simulink library "csc_cnt_attitude_control_lib_diag"  (R2015b)
settings: Solver=ode45  StartTime=0.0  StopTime=10.0  RelTol=1e-3
undefined symbols (not defined in the file or in its folder): csc_cnt_dt, gdn_altitude_transition_free_drift_landing, gdn_altitude_transition_free_drift_takeoff
libraries: util_quat_lib x3, util_common_lib x2, util_info_lib x1, util_extra_lib x1, csc_ppc_phase_plane_ctrl_lib_diag x1, csu_iqf_inertial_quat_feedback_lib x1
settings Model: Creator=ianmga  LastModifiedBy=jimkaidy
settings DataIOCC: SaveFormat=Array  SignalLoggingSaveFormat=ModelDataLogs
settings OptimizationCC: ExpressionDepthLimit=2147483647
settings DebuggingCC: UnderspecifiedInitializationDetection=Classic  MergeDetectMultiDrivingBlocksExec=none  SolverPrmCheckMsg=warning  FcnCallInpInsideContextMsg=UseLocalSettings  StateNameClashWarn=warning
settings HardwareCC: ProdBitPerPointer=32  ProdLargestAtomicFloat=None  ProdIntDivRoundTo=Undefined  ProdEndianess=Unspecified  ProdWordSize=32  ProdHWDeviceType=32-bit Generic
settings GRTTargetCC: GeneratePreprocessorConditionals=Disable all  CombineOutputUpdateFcns=off  GRTInterface=on
settings ConfigComp: CovModelRefEnable=Off  CovSFcnEnable=off

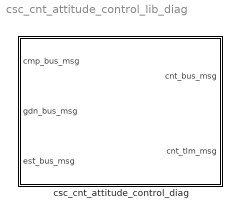
== system csc_cnt_attitude_control_lib_diag ==
  csc_cnt_attitude_control_diag : Subsystem  Tag=OFSW; MDL_TICK=GDN_BUS_MSG  TreatAsAtomicUnit=on  SystemSampleTime=csc_cnt_dt

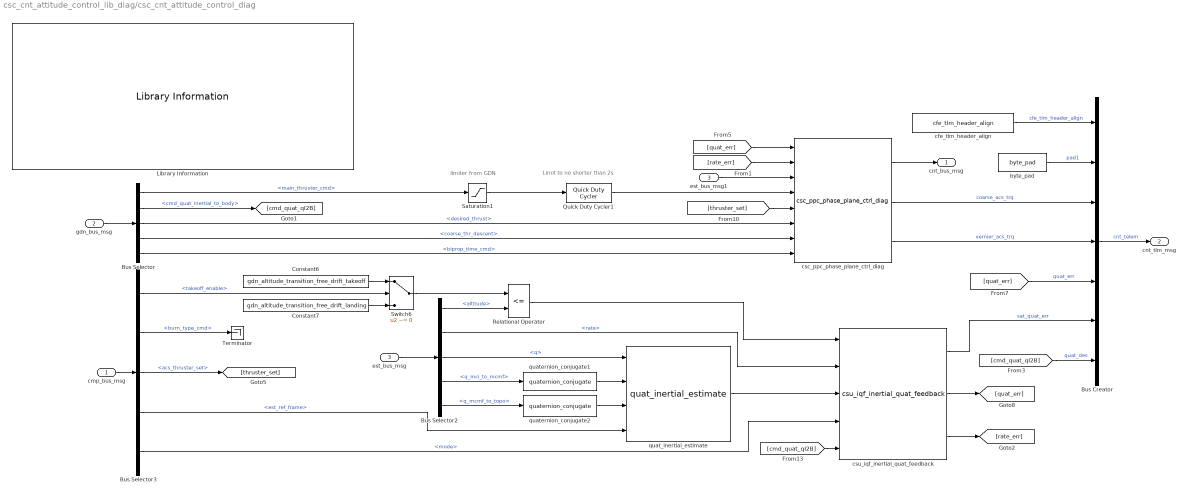
== system csc_cnt_attitude_control_lib_diag/csc_cnt_attitude_control_diag ==
  note: limiter from GDN
  note: Limit to no shorter than 2s
  cmp_bus_msg : Inport
  gdn_bus_msg : Inport  Port=2  OutDataTypeStr=Bus: gdn_bus_msg
  est_bus_msg : Inport  Port=3
  Bus Creator : BusCreator  Inputs=7  OutDataTypeStr=Bus: cnt_tlm_msg  NonVirtualBus=on
  Bus Selector2 : BusSelector  OutputSignals=altitude,rate,q,q_mci_to_mcmf,q_mcmf_to_topo
  Bus Selector3 : BusSelector  OutputSignals=takeoff_enable,burn_type_cmd,acs_thruster_set,est_ref_frame,mode
  Bus Selector : BusSelector  OutputSignals=main_thruster_cmd,cmd_quat_inertial_to_body,desired_thrust,coarse_thr_descent,biprop_time_cmd
  Constant6 : Constant  Value=gdn_altitude_transition_free_drift_takeoff  VectorParams1D=off
  Constant7 : Constant  Value=gdn_altitude_transition_free_drift_landing  VectorParams1D=off
  Library Information : util_info_lib/Library Information  owner='NONE'
  Quick Duty Cycler1 : util_extra_lib/Quick Duty Cycler  min_dt=2  dt=csc_cnt_dt
  Relational Operator : RelationalOperator  Operator=<=  OutDataTypeStr=boolean
  Saturation1 : Saturate  UpperLimit=1.1  LowerLimit=0.0
  Switch6 : Switch  Criteria=u2 ~= 0
  Terminator : Terminator
  byte_pad : util_common_lib/byte_pad  n_bytes=6
  cfe_tlm_header_align : util_common_lib/cfe_tlm_header_align
  csc_ppc_phase_plane_ctrl_diag : csc_ppc_phase_plane_ctrl_lib_diag/csc_ppc_phase_plane_ctrl_diag
  csu_iqf_inertial_quat_feedback : csu_iqf_inertial_quat_feedback_lib/csu_iqf_inertial_quat_feedback
  est_bus_msg1 : InportShadow  Port=3
  quat_inertial_estimate : util_quat_lib/quat_inertial_estimate  SystemSampleTime=-1
  quaternion_conjugate1 : util_quat_lib/quaternion_conjugate  SystemSampleTime=-1
  quaternion_conjugate2 : util_quat_lib/quaternion_conjugate  SystemSampleTime=-1
  cnt_bus_msg : Outport  OutDataTypeStr=Bus: cnt_bus_msg
  cnt_tlm_msg : Outport  Port=2  OutDataTypeStr=Bus: cnt_tlm_msg
  wires:
  [rate_err] -> csc_ppc_phase_plane_ctrl_diag/2
  csu_iqf_inertial_quat_feedback/3 -> [rate_err]
  Bus Selector2/2 -> csu_iqf_inertial_quat_feedback/2  "<rate>"
  cfe_tlm_header_align/1 -> Bus Creator/1  "cfe_tlm_header_align"
  quaternion_conjugate2/1 -> quat_inertial_estimate/3
  quaternion_conjugate1/1 -> quat_inertial_estimate/2
  Relational Operator/1 -> csu_iqf_inertial_quat_feedback/1
  csu_iqf_inertial_quat_feedback/1 -> Bus Creator/6  "sat_quat_err"
  Bus Selector3/4 -> quat_inertial_estimate/4  "<est_ref_frame>"
  Bus Selector2/1 -> Relational Operator/2  "<altitude>"
  Bus Selector2/5 -> quaternion_conjugate2/1  "<q_mcmf_to_topo>"
  Bus Selector2/4 -> quaternion_conjugate1/1  "<q_mci_to_mcmf>"
  quat_inertial_estimate/1 -> csu_iqf_inertial_quat_feedback/3
  csc_ppc_phase_plane_ctrl_diag/3 -> Bus Creator/4  "vernier_acs_trq"
  csc_ppc_phase_plane_ctrl_diag/2 -> Bus Creator/3  "coarse_acs_trq"
  Saturation1/1 -> Quick Duty Cycler1/1
  Bus Selector3/5 -> csu_iqf_inertial_quat_feedback/4  "<mode>"
  est_bus_msg1/1 -> csc_ppc_phase_plane_ctrl_diag/3
  Switch6/1 -> Relational Operator/1
  Bus Selector/4 -> csc_ppc_phase_plane_ctrl_diag/7  "<coarse_thr_descent>"
  [thruster_set] -> csc_ppc_phase_plane_ctrl_diag/5
  Bus Selector3/3 -> [thruster_set]  "<acs_thruster_set>"
  [quat_err] -> csc_ppc_phase_plane_ctrl_diag/1
  [cmd_quat_qI2B] -> csu_iqf_inertial_quat_feedback/5
  Bus Selector2/3 -> quat_inertial_estimate/1  "<q>"
  est_bus_msg/1 -> Bus Selector2/1
  Bus Selector3/2 -> Terminator/1  "<burn_type_cmd>"
  Bus Selector/1 -> Saturation1/1  "<main_thruster_cmd>"
  [cmd_quat_qI2B] -> Bus Creator/7  "quat_des"
  Bus Selector/2 -> [cmd_quat_qI2B]  "<cmd_quat_inertial_to_body>"
  Bus Creator/1 -> cnt_tlm_msg/1  "cnt_telem"
  gdn_bus_msg/1 -> Bus Selector/1
  [quat_err] -> Bus Creator/5  "quat_err"
  Bus Selector3/1 -> Switch6/2  "<takeoff_enable>"
  cmp_bus_msg/1 -> Bus Selector3/1
  Constant7/1 -> Switch6/3
  Constant6/1 -> Switch6/1
  csu_iqf_inertial_quat_feedback/2 -> [quat_err]
  csc_ppc_phase_plane_ctrl_diag/1 -> cnt_bus_msg/1
  Quick Duty Cycler1/1 -> csc_ppc_phase_plane_ctrl_diag/4
  byte_pad/1 -> Bus Creator/2  "pad1"
  Bus Selector/3 -> csc_ppc_phase_plane_ctrl_diag/6  "<desired_thrust>"
  Bus Selector/5 -> csc_ppc_phase_plane_ctrl_diag/8  "<biprop_time_cmd>"
